simulink model "PowertrainMaxPowerController"  (R2019b)
settings: Solver=ode4  StartTime=0.0  StopTime=inf  FixedStep=.01  RelTol=1e-3  EnableMultiTasking=on
model workspace (MAT data in the model file):
  CONVERTER_DATA = [0  137.465208994  2.232; 0.1  137.065019157  2.075; 0.2  135.864449646  1.975; 0.3  135.664354728  1.846; 0.4  137.565256453  1.72; 0.5  140.366585312  1.564; 0.6  145.268910814  1.409; 0.7  152.872517717  1.254; 0.8  162.9773111  1.096; 0.81  164.27792807  1.08; 0.82  166.178829795  1.061; 0.83  167.979684062  1.043; 0.84  170.080680706  1.028; 0.85  172.781962105  1.012; 0.86  175.383196045  1.002; 0.87  179.585189333  1.002; 0.88  183.587087703  1.001; 0.89  189.890077635  0.998; 0.9  197.693779455  0.999; 0.92  215.902417037  1.001; 0.94  244.515990379  1.002]
  DOWN_TABLE = [0  5  10  20  30; 0  5  10  20  30; 0  7.5  20  30  40; 0  7.5  20  30  40; 0  15  30  50  60; 0  15  30  50  60]
  DOWN_TH_BP = [0 5 40 50 90 100]
  EMAP = [-40  -44  -49  -53  -57  -61  -65  -70  -74  -78  -82; 215  117  85  66  44  29  10  -2  -13  -22  -32; 245  208  178  148  122  104  85  66  48  33  18; 264  260  241  219  193  167  152  133  119  96  85; 264  279  282  275  260  238  223  208  189  171  152; 267  290  293  297  290  275  260  256  234  212  193; 267  297  305  305  305  301  293  282  267  249  226; 267  301  308  312  319  323  319  316  297  279  253; 267  301  312  319  327  327  327  327  312  293  267; 267  301  312  319  327  334  334  334  319  305  275]
  NE_VEC = [800 1200 1600 2000 2400 2800 3200 3600 4000 4400 4800]
  TH_VEC = [0; 20; 30; 40; 50; 60; 70; 80; 90; 100]
  TWAITdn = 1.25
  TWAITup = 0.1
  Tin = [1  2; 2  2; 3  2; 4  2; 5  2; 6  0; 7  0; 8  0; 9  0; 10  0]
  UP_TABLE = [7.5  25  40  50  60; 7.5  25  40  50  60; 15  35  50  60  70; 25  45  60  70  80; 40  70  90  100  110; 40  80  90  100  110]
  UP_TH_BP = [0 25 35 50 90 100]
  reqTmaxT = [nan  nan  nan  nan  nan  nan  nan  nan; 0.285774810084  0.209689533834  0.17164689571  0.133604257585  0.0955616194602  nan  nan  nan; 0.647179872268  0.495009319769  0.41892404352  0.342838767271  0.266753491021  0.152625576647  nan  nan; nan  0.780329105704  0.66620119133  0.552073276956  0.437945362582  0.266753491021  0.152625576647  0.0955616194602; nan  nan  0.913478339141  0.761307786642  0.609137234143  0.380881405395  0.228710852897  0.152625576647; nan  nan  nan  0.970542296328  0.780329105704  0.495009319769  0.304796129146  0.209689533834; nan  nan  nan  nan  0.951520977265  0.609137234143  0.380881405395  0.266753491021; nan  nan  nan  nan  nan  0.723265148517  0.456966681645  0.323817448208; nan  nan  nan  nan  nan  0.837393062891  0.533051957894  0.380881405395; nan  nan  nan  nan  nan  0.951520977265  0.609137234143  0.437945362582; nan  nan  nan  nan  nan  nan  0.685222510393  0.495009319769; nan  nan  nan  nan  nan  nan  0.761307786642  0.552073276956; nan  nan  nan  nan  nan  nan  0.837393062891  0.609137234143; nan  nan  nan  nan  nan  nan  0.913478339141  0.66620119133; nan  nan  nan  nan  nan  nan  0.98956361539  0.723265148517; nan  nan  nan  nan  nan  nan  nan  0.780329105704; nan  nan  nan  nan  nan  nan  nan  0.837393062891; nan  nan  nan  nan  nan  nan  nan  0.894457020078; nan  nan  nan  nan  nan  nan  nan  0.951520977265; nan  nan  nan  nan  nan  nan  nan  nan; nan  nan  nan  nan  nan  nan  nan  nan]
  vehSpd = [0 2.77777777778 5.55555555556 8.33333333333 11.1111111111 13.8888888889 16.6666666667 19.4444444444 22.2222222222 25 27.7777777778 30.5555555556 33.3333333333 36.1111111111 38.8888888889 41.6666666667 44.4444444444 47.2222222222 50 52.7777777778 55.5555555556]
settings Model: ModifiedByFormat=The MathWorks, Inc.  Creator=The MathWorks, Inc.  LastModifiedBy=The MathWorks, Inc.
settings DataIOCC: DSMLogging=off  ReturnWorkspaceOutputs=off
settings DebuggingCC: ArithmeticOperatorsInVariantConditions=warning
settings SFSimCC: SimUseLocalCustomCode=off  CustomCodeUndefinedFunction=UseInterfaceOnly
settings RTWCC: RTWUseLocalCustomCode=off
settings CodeAppCC: StateflowObjectComments=on
settings GRTTargetCC: TargetLangStandard=C89/C90 (ANSI)
settings ConfigComp: CovMetricSettings=dsw  CovHtmlReporting=on  CovSaveCumulativeToWorkspaceVar=on  CovSaveSingleToWorkspaceVar=on  CovShowResultsExplorer=off  CovExternalEMLEnable=off

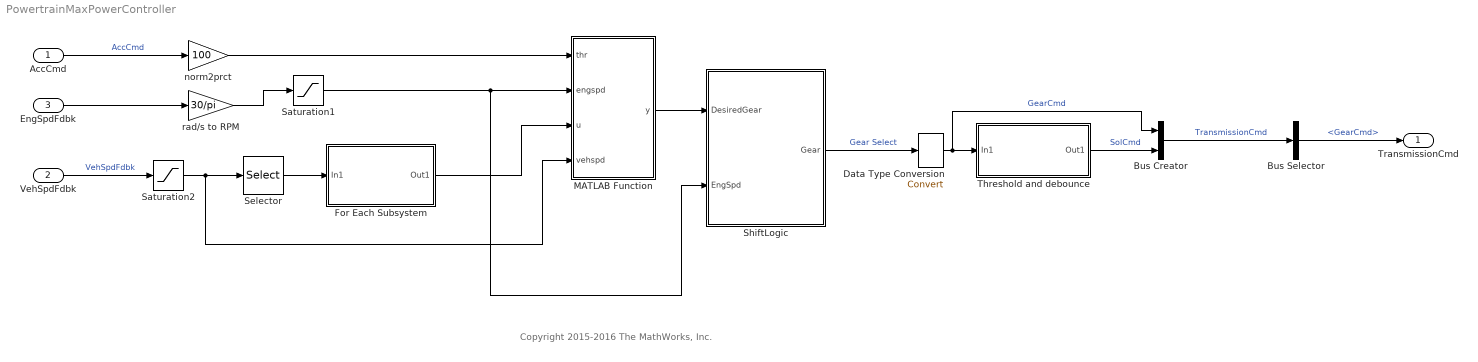
== system PowertrainMaxPowerController ==
  note: Copyright 2015-2016 The MathWorks, Inc.
  AccCmd : Inport
  VehSpdFdbk : Inport  Port=2
  EngSpdFdbk : Inport  Port=3
  Bus Creator : BusCreator  Inputs=2
  Bus Selector : BusSelector  OutputSignals=GearCmd
  Data Type Conversion : DataTypeConversion
  For Each Subsystem : Subsystem  TreatAsAtomicUnit=on  mask{breakPoints=vehSpd, tableData=reqTmaxT'}
      mask prompts: breakPoints "Break Points"; tableData "Table Data"
  MATLAB Function : MATLAB Function  TreatAsAtomicUnit=on
  Saturation1 : Saturate  UpperLimit=10e3  LowerLimit=0
  Saturation2 : Saturate  UpperLimit=200  LowerLimit=0
  Selector : Selector  InputPortWidth=1  IndexOptions=Index vector (dialog)  Indices=ones(8,1)  OutputSizes=1
  ShiftLogic : Stateflow chart  TreatAsAtomicUnit=on
  Threshold and debounce : Subsystem
  norm2prct : Gain  Gain=100
  rad/s to RPM : Gain  Gain=30/pi
  TransmissionCmd : Outport
  wires:
  AccCmd/1 -> norm2prct/1  "AccCmd"
  Selector/1 -> For Each Subsystem/1(In1)
  MATLAB Function/1(y) -> ShiftLogic/1(DesiredGear)
  norm2prct/1 -> MATLAB Function/1(thr)
  EngSpdFdbk/1 -> rad/s to RPM/1
  Saturation1/1 -> ShiftLogic/2(EngSpd), MATLAB Function/2(engspd)
  ShiftLogic/1(Gear) -> Data Type Conversion/1  "Gear Select"
  Threshold and debounce/1(Out1) -> Bus Creator/2  "SolCmd"
  Data Type Conversion/1 -> Bus Creator/1, Threshold and debounce/1(In1)  "GearCmd"
  Bus Creator/1 -> Bus Selector/1  "TransmissionCmd"
  Bus Selector/1 -> TransmissionCmd/1  "<GearCmd>"
  rad/s to RPM/1 -> Saturation1/1
  Saturation2/1 -> MATLAB Function/4(vehspd), Selector/1
  VehSpdFdbk/1 -> Saturation2/1  "VehSpdFdbk"
  For Each Subsystem/1(Out1) -> MATLAB Function/3(u)

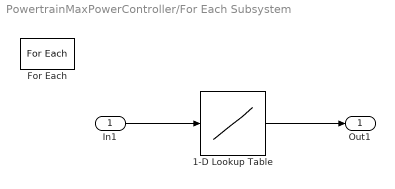
== system PowertrainMaxPowerController/For Each Subsystem ==
  In1 : Inport  Partition=on  PartitionDimension=1  PartitionWidth=1  PartitionOffset=0
  1-D Lookup Table : Lookup_n-D  NumberOfTableDimensions=1  LookupTableObject=''  BreakpointsForDimension1=breakPoints  Table=tableData  ExtrapMethod=Clip  UseLastTableValue=on  InternalRulePriority=Speed  RndMeth=Simplest  InputSameDT=on
  For Each : ForEach  DisableCoverage=on  IterateSubsysMaskParameter=off,on
  Out1 : Outport  ConcatenationDimension=1
  wires:
  In1/1 -> 1-D Lookup Table/1
  1-D Lookup Table/1 -> Out1/1

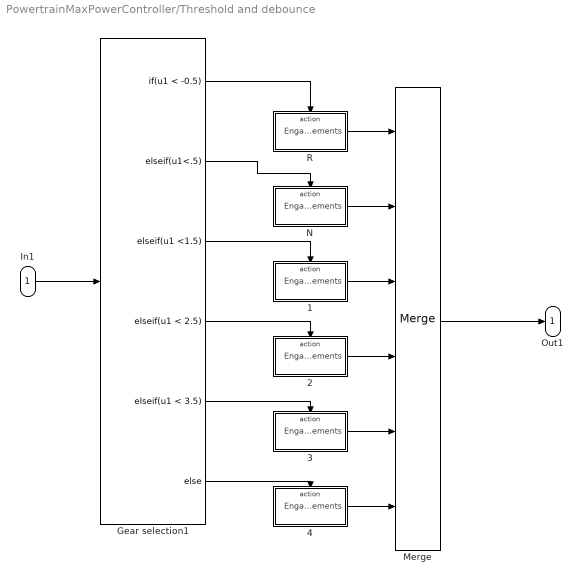
== system PowertrainMaxPowerController/Threshold and debounce ==
  In1 : Inport
  1 : Subsystem  TreatAsAtomicUnit=on
  2 : Subsystem  TreatAsAtomicUnit=on
  3 : Subsystem  TreatAsAtomicUnit=on
  4 : Subsystem  TreatAsAtomicUnit=on
  Gear selection1 : If  IfExpression=u1 < -0.5  ElseIfExpressions=u1<.5, u1 <1.5, u1 < 2.5, u1 < 3.5
  Merge : Merge  Inputs=6
  N : Subsystem  TreatAsAtomicUnit=on
  R : Subsystem  TreatAsAtomicUnit=on
  Out1 : Outport
  wires:
  N/1(Engagements) -> Merge/2
  Gear selection1/2 -> N/Action
  Gear selection1/6 -> 4/Action
  4/1(Engagements) -> Merge/6
  1/1(Engagements) -> Merge/3
  3/1(Engagements) -> Merge/5
  2/1(Engagements) -> Merge/4
  R/1(Engagements) -> Merge/1
  Gear selection1/5 -> 3/Action
  Gear selection1/4 -> 2/Action
  Gear selection1/3 -> 1/Action
  Gear selection1/1 -> R/Action
  In1/1 -> Gear selection1/1
  Merge/1 -> Out1/1

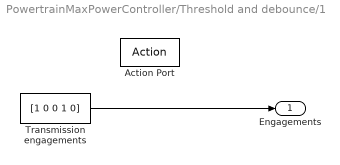
== system PowertrainMaxPowerController/Threshold and debounce/1 ==
  Action Port : ActionPort  ActionPortLabel=elseif { }
  Transmission engagements : Constant  Value=[1 0 0 1 0]
  Engagements : Outport  InitialOutput=[0, 0, 0, 0, 0]
  wires:
  Transmission engagements/1 -> Engagements/1

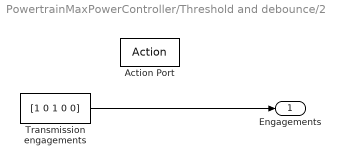
== system PowertrainMaxPowerController/Threshold and debounce/2 ==
  Action Port : ActionPort  ActionPortLabel=elseif { }
  Transmission engagements : Constant  Value=[1 0 1 0 0]
  Engagements : Outport  InitialOutput=[0, 0, 0, 0, 0]
  wires:
  Transmission engagements/1 -> Engagements/1

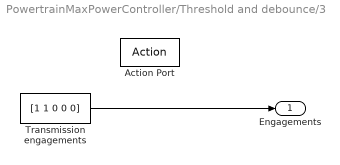
== system PowertrainMaxPowerController/Threshold and debounce/3 ==
  Action Port : ActionPort  ActionPortLabel=elseif { }
  Transmission engagements : Constant  Value=[1 1 0 0 0]
  Engagements : Outport  InitialOutput=[0, 0, 0, 0, 0]
  wires:
  Transmission engagements/1 -> Engagements/1

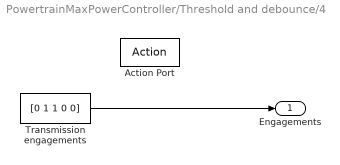
== system PowertrainMaxPowerController/Threshold and debounce/4 ==
  Action Port : ActionPort  ActionPortLabel=else { }
  Transmission engagements : Constant  Value=[0 1 1 0 0]
  Engagements : Outport  InitialOutput=[0, 0, 0, 0, 0]
  wires:
  Transmission engagements/1 -> Engagements/1

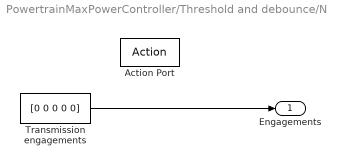
== system PowertrainMaxPowerController/Threshold and debounce/N ==
  Action Port : ActionPort  ActionPortLabel=elseif { }
  Transmission engagements : Constant  Value=[0 0 0 0 0]
  Engagements : Outport  InitialOutput=[0, 0, 0, 0, 0]
  wires:
  Transmission engagements/1 -> Engagements/1

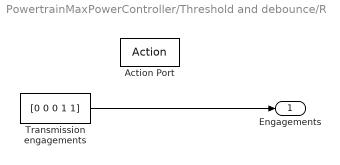
== system PowertrainMaxPowerController/Threshold and debounce/R ==
  Action Port : ActionPort  ActionPortLabel=if { }
  Transmission engagements : Constant  Value=[0 0 0 1 1]
  Engagements : Outport  InitialOutput=[0, 0, 0, 0, 0]
  wires:
  Transmission engagements/1 -> Engagements/1

== matlab function PowertrainMaxPowerController/MATLAB Function ==
  data: thr input; engspd input; u input; vehspd input; y output
function y = fcn(thr,engspd,u,vehspd)

if ((thr<1)&&(vehspd<5))||(engspd<600)
    y=0;
else
   [~, y] = max(u);
end

== stateflow chart PowertrainMaxPowerController/ShiftLogic ==
  settings: updateMethod=DISCRETE  sampleTime=0.01
  state gear_state [parallel]
    settings: executionOrder=1
    state even
    state neutral
      entry:
      Gear = 0;
    state odd
    (junction 75) -> (junction 76)
    (junction 76) -> odd
    even -> (junction 75) [order 1] : UP
        | {Gear=Gear+1;}
    (default) -> neutral
    odd -> even [order 1] : UP
        | {Gear=Gear+1;}
    neutral -> odd : UP
        | {Gear=Gear+1;}
    even -> odd [order 2] : DOWN
        | {Gear=Gear-1;}
    (junction 87) -> even
    even -> (junction 91) [order 3] : [Gear==0]
    odd -> (junction 85) [order 2] : DOWN
        | {Gear=Gear-1;}
    (junction 93) -> neutral
    (junction 85) -> (junction 87)
    (junction 91) -> (junction 93)
  state selection_state [parallel]
    settings: executionOrder=2
    state steady_state
    state upshifting
    state downshifting
    (default) -> steady_state
    steady_state -> upshifting [order 1] : [DesiredGear> Gear]
    steady_state -> downshifting [order 2] : [DesiredGear < Gear]
    downshifting -> steady_state [order 3] : [EngSpd<1000.]{gear_state.DOWN;}
    downshifting -> steady_state [order 1] : after(TWAITdn,sec)
        | {gear_state.DOWN;}
    downshifting -> steady_state [order 2] : [Gear == DesiredGear]
    upshifting -> steady_state [order 1] : after(TWAITup,sec)
        | {gear_state.UP;}
    upshifting -> steady_state [order 2] : [Gear == DesiredGear]
  data: Gear output int8 [1..4]; TWAITdn parameter double; DesiredGear input; TWAITup parameter double; EngSpd input
  events: DOWN local EITHER_EDGE_EVENT; UP local EITHER_EDGE_EVENT
